simulink library "myLibrary"  (R2023a)
settings: Solver=VariableStepAuto  StartTime=0.0  StopTime=10.0  RelTol=1e-3
undefined symbols (not defined in the file): Cac_n1, ctrl1, Da, Discrete, dtha, ee_sli_rtmsupport, FA, gcbh, Ha, Ini, init_line, init_load, init_SG, init_TH, init_trafo, init_VSC, initMachineBlocks, Ka, Lf, Llkd_pu, Llkq1_pu, NET, P, plots_step, q0, Rac_n1, Radd, Rkd_pu, Rkq1_pu, Rload_add, sim_config, spsSteamTurbineModel, T_global, T_load, T_NET, T_SG, T_TH, T_trafo, T_VSC, Ts, tstep, V1
libraries: spsSeriesRLCBranchLib x57, spsParallelRLCBranchLib x39, eeGeneralControl x38, spsCurrentMeasurementLib x20, spsFirstOrderFilterLib x16, spsVoltageMeasurementLib x14, spsControlledVoltageSourceLib x12, $bdroot x9, dspsigops x6, spsThreePhaseVIMeasurementLib x5, spsPLL3phLib x4, spsThreePhaseBreakerLib x3
(part 5 of 7)

== system myLibrary/GFOL/Control/Is3/Matriu T ==
  u : Inport
  Constant : Constant  Value=(2/3)*[1/2 1/2 1/2]
  Fcn : Fcn  Expr=(2/3)*cos(u)
  Fcn1 : Fcn  Expr=(2/3)*cos(u-(2*pi)/3)
  Fcn2 : Fcn  Expr=(2/3)*cos(u+(2*pi)/3)
  Fcn3 : Fcn  Expr=(2/3)*sin(u)
  Fcn4 : Fcn  Expr=(2/3)*sin(u-(2*pi)/3)
  Fcn5 : Fcn  Expr=(2/3)*sin(u+(2*pi)/3)
  Math Function : Math  Operator=transpose  SignedPower=on
  Matrix Concatenate : Concatenate  NumInputs=3  Mode=Multidimensional array  ConcatenateDimension=2
  Mux : Mux  Inputs=3
  Mux1 : Mux  Inputs=3
  Out1 : Outport  VectorParamsAs1DForOutWhenUnconnected=off
  wires:
  u/1 -> Fcn/1, Fcn1/1, Fcn2/1, Fcn3/1, Fcn4/1, Fcn5/1
  Fcn3/1 -> Mux1/1
  Fcn4/1 -> Mux1/2
  Fcn5/1 -> Mux1/3
  Mux/1 -> Matrix Concatenate/1
  Constant/1 -> Matrix Concatenate/3
  Fcn/1 -> Mux/1
  Fcn1/1 -> Mux/2
  Fcn2/1 -> Mux/3
  Mux1/1 -> Matrix Concatenate/2
  Matrix Concatenate/1 -> Math Function/1
  Math Function/1 -> Out1/1

== system myLibrary/GFOL/Control/Is4/Matriu T ==
  u : Inport
  Constant : Constant  Value=(2/3)*[1/2 1/2 1/2]
  Fcn : Fcn  Expr=(2/3)*cos(u)
  Fcn1 : Fcn  Expr=(2/3)*cos(u-(2*pi)/3)
  Fcn2 : Fcn  Expr=(2/3)*cos(u+(2*pi)/3)
  Fcn3 : Fcn  Expr=(2/3)*sin(u)
  Fcn4 : Fcn  Expr=(2/3)*sin(u-(2*pi)/3)
  Fcn5 : Fcn  Expr=(2/3)*sin(u+(2*pi)/3)
  Math Function : Math  Operator=transpose  SignedPower=on
  Matrix Concatenate : Concatenate  NumInputs=3  Mode=Multidimensional array  ConcatenateDimension=2
  Mux : Mux  Inputs=3
  Mux1 : Mux  Inputs=3
  Out1 : Outport  VectorParamsAs1DForOutWhenUnconnected=off
  wires:
  Math Function/1 -> Out1/1
  Matrix Concatenate/1 -> Math Function/1
  Mux1/1 -> Matrix Concatenate/2
  Fcn2/1 -> Mux/3
  Fcn1/1 -> Mux/2
  Fcn/1 -> Mux/1
  Constant/1 -> Matrix Concatenate/3
  Mux/1 -> Matrix Concatenate/1
  Fcn5/1 -> Mux1/3
  Fcn4/1 -> Mux1/2
  Fcn3/1 -> Mux1/1
  u/1 -> Fcn5/1, Fcn4/1, Fcn3/1, Fcn2/1, Fcn1/1, Fcn/1

== system myLibrary/GFOL/Control/Is5/Matriu T ==
  u : Inport
  Constant : Constant  Value=(2/3)*[1/2 1/2 1/2]
  Fcn : Fcn  Expr=(2/3)*cos(u)
  Fcn1 : Fcn  Expr=(2/3)*cos(u-(2*pi)/3)
  Fcn2 : Fcn  Expr=(2/3)*cos(u+(2*pi)/3)
  Fcn3 : Fcn  Expr=(2/3)*sin(u)
  Fcn4 : Fcn  Expr=(2/3)*sin(u-(2*pi)/3)
  Fcn5 : Fcn  Expr=(2/3)*sin(u+(2*pi)/3)
  Math Function : Math  Operator=transpose  SignedPower=on
  Matrix Concatenate : Concatenate  NumInputs=3  Mode=Multidimensional array  ConcatenateDimension=2
  Mux : Mux  Inputs=3
  Mux1 : Mux  Inputs=3
  Out1 : Outport  VectorParamsAs1DForOutWhenUnconnected=off
  wires:
  u/1 -> Fcn/1, Fcn1/1, Fcn2/1, Fcn3/1, Fcn4/1, Fcn5/1
  Fcn3/1 -> Mux1/1
  Fcn4/1 -> Mux1/2
  Fcn5/1 -> Mux1/3
  Mux/1 -> Matrix Concatenate/1
  Constant/1 -> Matrix Concatenate/3
  Fcn/1 -> Mux/1
  Fcn1/1 -> Mux/2
  Fcn2/1 -> Mux/3
  Mux1/1 -> Matrix Concatenate/2
  Matrix Concatenate/1 -> Math Function/1
  Math Function/1 -> Out1/1

== system myLibrary/GFOL/Control/Is7/Matriu T ==
  u : Inport
  Constant : Constant  Value=(2/3)*[1/2 1/2 1/2]
  Fcn : Fcn  Expr=(2/3)*cos(u)
  Fcn1 : Fcn  Expr=(2/3)*cos(u-(2*pi)/3)
  Fcn2 : Fcn  Expr=(2/3)*cos(u+(2*pi)/3)
  Fcn3 : Fcn  Expr=(2/3)*sin(u)
  Fcn4 : Fcn  Expr=(2/3)*sin(u-(2*pi)/3)
  Fcn5 : Fcn  Expr=(2/3)*sin(u+(2*pi)/3)
  Math Function : Math  Operator=transpose  SignedPower=on
  Matrix Concatenate : Concatenate  NumInputs=3  Mode=Multidimensional array  ConcatenateDimension=2
  Mux : Mux  Inputs=3
  Mux1 : Mux  Inputs=3
  Out1 : Outport  VectorParamsAs1DForOutWhenUnconnected=off
  wires:
  Math Function/1 -> Out1/1
  Matrix Concatenate/1 -> Math Function/1
  Mux1/1 -> Matrix Concatenate/2
  Fcn2/1 -> Mux/3
  Fcn1/1 -> Mux/2
  Fcn/1 -> Mux/1
  Constant/1 -> Matrix Concatenate/3
  Mux/1 -> Matrix Concatenate/1
  Fcn5/1 -> Mux1/3
  Fcn4/1 -> Mux1/2
  Fcn3/1 -> Mux1/1
  u/1 -> Fcn5/1, Fcn4/1, Fcn3/1, Fcn2/1, Fcn1/1, Fcn/1

== system myLibrary/GFOL/Control/PLL/Tpark ==
  Va : Inport
  Vb : Inport  Port=2
  Vc : Inport  Port=3
  u : Inport  Port=4
  Demux : Demux  Outputs=3
  Matriu T : Subsystem
  Mux : Mux  Inputs=3
      settings: DisplayOption=signals
  Product : Product  Multiplication=Matrix(*)
  Vq : Outport  VectorParamsAs1DForOutWhenUnconnected=off
  Vd : Outport  Port=2  VectorParamsAs1DForOutWhenUnconnected=off
  0 : Outport  Port=3  VectorParamsAs1DForOutWhenUnconnected=off
  wires:
  Matriu T/1(Out1) -> Product/1
  Mux/1 -> Product/2
  u/1 -> Matriu T/1(u)
  Demux/3 -> 0/1
  Demux/2 -> Vd/1
  Demux/1 -> Vq/1
  Product/1 -> Demux/1
  Vc/1 -> Mux/3
  Vb/1 -> Mux/2
  Va/1 -> Mux/1

== system myLibrary/GFOL_RL/Control/Is/Matriu T ==
  u : Inport
  Constant : Constant  Value=(2/3)*[1/2 1/2 1/2]
  Fcn : Fcn  Expr=(2/3)*cos(u)
  Fcn1 : Fcn  Expr=(2/3)*cos(u-(2*pi)/3)
  Fcn2 : Fcn  Expr=(2/3)*cos(u+(2*pi)/3)
  Fcn3 : Fcn  Expr=(2/3)*sin(u)
  Fcn4 : Fcn  Expr=(2/3)*sin(u-(2*pi)/3)
  Fcn5 : Fcn  Expr=(2/3)*sin(u+(2*pi)/3)
  Math Function : Math  Operator=transpose  SignedPower=on
  Matrix Concatenate : Concatenate  NumInputs=3  Mode=Multidimensional array  ConcatenateDimension=2
  Mux : Mux  Inputs=3
  Mux1 : Mux  Inputs=3
  Out1 : Outport  VectorParamsAs1DForOutWhenUnconnected=off
  wires:
  u/1 -> Fcn/1, Fcn1/1, Fcn2/1, Fcn3/1, Fcn4/1, Fcn5/1
  Fcn3/1 -> Mux1/1
  Fcn4/1 -> Mux1/2
  Fcn5/1 -> Mux1/3
  Mux/1 -> Matrix Concatenate/1
  Constant/1 -> Matrix Concatenate/3
  Fcn/1 -> Mux/1
  Fcn1/1 -> Mux/2
  Fcn2/1 -> Mux/3
  Mux1/1 -> Matrix Concatenate/2
  Matrix Concatenate/1 -> Math Function/1
  Math Function/1 -> Out1/1

== system myLibrary/GFOL_RL/Control/Is1/Matriu T ==
  u : Inport
  Constant : Constant  Value=(2/3)*[1/2 1/2 1/2]
  Fcn : Fcn  Expr=(2/3)*cos(u)
  Fcn1 : Fcn  Expr=(2/3)*cos(u-(2*pi)/3)
  Fcn2 : Fcn  Expr=(2/3)*cos(u+(2*pi)/3)
  Fcn3 : Fcn  Expr=(2/3)*sin(u)
  Fcn4 : Fcn  Expr=(2/3)*sin(u-(2*pi)/3)
  Fcn5 : Fcn  Expr=(2/3)*sin(u+(2*pi)/3)
  Math Function : Math  Operator=transpose  SignedPower=on
  Matrix Concatenate : Concatenate  NumInputs=3  Mode=Multidimensional array  ConcatenateDimension=2
  Mux : Mux  Inputs=3
  Mux1 : Mux  Inputs=3
  Out1 : Outport  VectorParamsAs1DForOutWhenUnconnected=off
  wires:
  Math Function/1 -> Out1/1
  Matrix Concatenate/1 -> Math Function/1
  Mux1/1 -> Matrix Concatenate/2
  Fcn2/1 -> Mux/3
  Fcn1/1 -> Mux/2
  Fcn/1 -> Mux/1
  Constant/1 -> Matrix Concatenate/3
  Mux/1 -> Matrix Concatenate/1
  Fcn5/1 -> Mux1/3
  Fcn4/1 -> Mux1/2
  Fcn3/1 -> Mux1/1
  u/1 -> Fcn5/1, Fcn4/1, Fcn3/1, Fcn2/1, Fcn1/1, Fcn/1

== system myLibrary/GFOL_RL/Control/Is3/Matriu T ==
  u : Inport
  Constant : Constant  Value=(2/3)*[1/2 1/2 1/2]
  Fcn : Fcn  Expr=(2/3)*cos(u)
  Fcn1 : Fcn  Expr=(2/3)*cos(u-(2*pi)/3)
  Fcn2 : Fcn  Expr=(2/3)*cos(u+(2*pi)/3)
  Fcn3 : Fcn  Expr=(2/3)*sin(u)
  Fcn4 : Fcn  Expr=(2/3)*sin(u-(2*pi)/3)
  Fcn5 : Fcn  Expr=(2/3)*sin(u+(2*pi)/3)
  Math Function : Math  Operator=transpose  SignedPower=on
  Matrix Concatenate : Concatenate  NumInputs=3  Mode=Multidimensional array  ConcatenateDimension=2
  Mux : Mux  Inputs=3
  Mux1 : Mux  Inputs=3
  Out1 : Outport  VectorParamsAs1DForOutWhenUnconnected=off
  wires:
  u/1 -> Fcn/1, Fcn1/1, Fcn2/1, Fcn3/1, Fcn4/1, Fcn5/1
  Fcn3/1 -> Mux1/1
  Fcn4/1 -> Mux1/2
  Fcn5/1 -> Mux1/3
  Mux/1 -> Matrix Concatenate/1
  Constant/1 -> Matrix Concatenate/3
  Fcn/1 -> Mux/1
  Fcn1/1 -> Mux/2
  Fcn2/1 -> Mux/3
  Mux1/1 -> Matrix Concatenate/2
  Matrix Concatenate/1 -> Math Function/1
  Math Function/1 -> Out1/1

== system myLibrary/GFOL_RL/Control/Is4/Matriu T ==
  u : Inport
  Constant : Constant  Value=(2/3)*[1/2 1/2 1/2]
  Fcn : Fcn  Expr=(2/3)*cos(u)
  Fcn1 : Fcn  Expr=(2/3)*cos(u-(2*pi)/3)
  Fcn2 : Fcn  Expr=(2/3)*cos(u+(2*pi)/3)
  Fcn3 : Fcn  Expr=(2/3)*sin(u)
  Fcn4 : Fcn  Expr=(2/3)*sin(u-(2*pi)/3)
  Fcn5 : Fcn  Expr=(2/3)*sin(u+(2*pi)/3)
  Math Function : Math  Operator=transpose  SignedPower=on
  Matrix Concatenate : Concatenate  NumInputs=3  Mode=Multidimensional array  ConcatenateDimension=2
  Mux : Mux  Inputs=3
  Mux1 : Mux  Inputs=3
  Out1 : Outport  VectorParamsAs1DForOutWhenUnconnected=off
  wires:
  Math Function/1 -> Out1/1
  Matrix Concatenate/1 -> Math Function/1
  Mux1/1 -> Matrix Concatenate/2
  Fcn2/1 -> Mux/3
  Fcn1/1 -> Mux/2
  Fcn/1 -> Mux/1
  Constant/1 -> Matrix Concatenate/3
  Mux/1 -> Matrix Concatenate/1
  Fcn5/1 -> Mux1/3
  Fcn4/1 -> Mux1/2
  Fcn3/1 -> Mux1/1
  u/1 -> Fcn5/1, Fcn4/1, Fcn3/1, Fcn2/1, Fcn1/1, Fcn/1

== system myLibrary/GFOL_RL/Control/Is5/Matriu T ==
  u : Inport
  Constant : Constant  Value=(2/3)*[1/2 1/2 1/2]
  Fcn : Fcn  Expr=(2/3)*cos(u)
  Fcn1 : Fcn  Expr=(2/3)*cos(u-(2*pi)/3)
  Fcn2 : Fcn  Expr=(2/3)*cos(u+(2*pi)/3)
  Fcn3 : Fcn  Expr=(2/3)*sin(u)
  Fcn4 : Fcn  Expr=(2/3)*sin(u-(2*pi)/3)
  Fcn5 : Fcn  Expr=(2/3)*sin(u+(2*pi)/3)
  Math Function : Math  Operator=transpose  SignedPower=on
  Matrix Concatenate : Concatenate  NumInputs=3  Mode=Multidimensional array  ConcatenateDimension=2
  Mux : Mux  Inputs=3
  Mux1 : Mux  Inputs=3
  Out1 : Outport  VectorParamsAs1DForOutWhenUnconnected=off
  wires:
  u/1 -> Fcn/1, Fcn1/1, Fcn2/1, Fcn3/1, Fcn4/1, Fcn5/1
  Fcn3/1 -> Mux1/1
  Fcn4/1 -> Mux1/2
  Fcn5/1 -> Mux1/3
  Mux/1 -> Matrix Concatenate/1
  Constant/1 -> Matrix Concatenate/3
  Fcn/1 -> Mux/1
  Fcn1/1 -> Mux/2
  Fcn2/1 -> Mux/3
  Mux1/1 -> Matrix Concatenate/2
  Matrix Concatenate/1 -> Math Function/1
  Math Function/1 -> Out1/1

== system myLibrary/GFOL_RL/Control/PLL/Tpark ==
  Va : Inport
  Vb : Inport  Port=2
  Vc : Inport  Port=3
  u : Inport  Port=4
  Demux : Demux  Outputs=3
  Matriu T : Subsystem
  Mux : Mux  Inputs=3
      settings: DisplayOption=signals
  Product : Product  Multiplication=Matrix(*)
  Vq : Outport  VectorParamsAs1DForOutWhenUnconnected=off
  Vd : Outport  Port=2  VectorParamsAs1DForOutWhenUnconnected=off
  0 : Outport  Port=3  VectorParamsAs1DForOutWhenUnconnected=off
  wires:
  Matriu T/1(Out1) -> Product/1
  Mux/1 -> Product/2
  u/1 -> Matriu T/1(u)
  Demux/3 -> 0/1
  Demux/2 -> Vd/1
  Demux/1 -> Vq/1
  Product/1 -> Demux/1
  Vc/1 -> Mux/3
  Vb/1 -> Mux/2
  Va/1 -> Mux/1

== system myLibrary/GFOR/Control/Is/Matriu T ==
  u : Inport
  Constant : Constant  Value=(2/3)*[1/2 1/2 1/2]
  Fcn : Fcn  Expr=(2/3)*cos(u)
  Fcn1 : Fcn  Expr=(2/3)*cos(u-(2*pi)/3)
  Fcn2 : Fcn  Expr=(2/3)*cos(u+(2*pi)/3)
  Fcn3 : Fcn  Expr=(2/3)*sin(u)
  Fcn4 : Fcn  Expr=(2/3)*sin(u-(2*pi)/3)
  Fcn5 : Fcn  Expr=(2/3)*sin(u+(2*pi)/3)
  Math Function : Math  Operator=transpose  SignedPower=on
  Matrix Concatenate : Concatenate  NumInputs=3  Mode=Multidimensional array  ConcatenateDimension=2
  Mux : Mux  Inputs=3
  Mux1 : Mux  Inputs=3
  Out1 : Outport  VectorParamsAs1DForOutWhenUnconnected=off
  wires:
  Math Function/1 -> Out1/1
  Matrix Concatenate/1 -> Math Function/1
  Mux1/1 -> Matrix Concatenate/2
  Fcn2/1 -> Mux/3
  Fcn1/1 -> Mux/2
  Fcn/1 -> Mux/1
  Constant/1 -> Matrix Concatenate/3
  Mux/1 -> Matrix Concatenate/1
  Fcn5/1 -> Mux1/3
  Fcn4/1 -> Mux1/2
  Fcn3/1 -> Mux1/1
  u/1 -> Fcn5/1, Fcn4/1, Fcn3/1, Fcn2/1, Fcn1/1, Fcn/1

== system myLibrary/GFOR/Control/Is2/Matriu T ==
  u : Inport
  Constant : Constant  Value=(2/3)*[1/2 1/2 1/2]
  Fcn : Fcn  Expr=(2/3)*cos(u)
  Fcn1 : Fcn  Expr=(2/3)*cos(u-(2*pi)/3)
  Fcn2 : Fcn  Expr=(2/3)*cos(u+(2*pi)/3)
  Fcn3 : Fcn  Expr=(2/3)*sin(u)
  Fcn4 : Fcn  Expr=(2/3)*sin(u-(2*pi)/3)
  Fcn5 : Fcn  Expr=(2/3)*sin(u+(2*pi)/3)
  Math Function : Math  Operator=transpose  SignedPower=on
  Matrix Concatenate : Concatenate  NumInputs=3  Mode=Multidimensional array  ConcatenateDimension=2
  Mux : Mux  Inputs=3
  Mux1 : Mux  Inputs=3
  Out1 : Outport  VectorParamsAs1DForOutWhenUnconnected=off
  wires:
  Math Function/1 -> Out1/1
  Matrix Concatenate/1 -> Math Function/1
  Mux1/1 -> Matrix Concatenate/2
  Fcn2/1 -> Mux/3
  Fcn1/1 -> Mux/2
  Fcn/1 -> Mux/1
  Constant/1 -> Matrix Concatenate/3
  Mux/1 -> Matrix Concatenate/1
  Fcn5/1 -> Mux1/3
  Fcn4/1 -> Mux1/2
  Fcn3/1 -> Mux1/1
  u/1 -> Fcn5/1, Fcn4/1, Fcn3/1, Fcn2/1, Fcn1/1, Fcn/1

== system myLibrary/SG/Exciter/Exciter ST4B/Fex ==
  V_E : Inport
  Ifd : Inport  Port=2
  Data Type Conversion Inherited : simulink/Signal Attributes/Data Type Conversion Inherited  ConvertRealWorld=Real World Value  DoSatur=off
  Divide : Product  Inputs=*/
  Gain : Gain  Gain=K_C  OutDataTypeStr=double
  Prevent divide by zero : Fcn  Expr=u+(u==0)*eps
  fex : MATLAB Function  TreatAsAtomicUnit=on
  F_EX : Outport  VectorParamsAs1DForOutWhenUnconnected=off
  wires:
  Data Type Conversion Inherited/1 -> F_EX/1
  fex/1(F_EX) -> Data Type Conversion Inherited/2  "F_EX"
  Gain/1 -> fex/1(I_N)  "I_N"
  Divide/1 -> Gain/1
  V_E/1 -> Prevent divide by zero/1
  Ifd/1 -> Divide/1, Data Type Conversion Inherited/1
  Prevent divide by zero/1 -> Divide/2

== system myLibrary/SG/Exciter/Exciter ST4B/PI_M ==
  u : Inport
  Constant2 : Constant  Value=0
  Gain2 : Gain  Gain=K_PM
  Gain3 : Gain  Gain=K_IM
  Integrator (Discrete or Continuous) : eeGeneralControl/Integrator (Discrete or Continuous)  LabelModeActiveChoice=Discrete  ExternalReset=level  LimitType=Anti-windup  B=inf  A=-inf  Ts=Ts
  Sum6 : Sum
  y : Outport
  wires:
  Gain3/1 -> Integrator (Discrete or Continuous)/1, Integrator (Discrete or Continuous)/3
  u/1 -> Gain2/1, Gain3/1
  Constant2/1 -> Integrator (Discrete or Continuous)/2
  Integrator (Discrete or Continuous)/1 -> Sum6/2
  Gain2/1 -> Sum6/1
  Sum6/1 -> y/1

== system myLibrary/SG/Exciter/Exciter ST4B/PI_R ==
  u : Inport
  Constant2 : Constant  Value=0
  Gain2 : Gain  Gain=K_PR
  Gain3 : Gain  Gain=K_IR
  Integrator (Discrete or Continuous) : eeGeneralControl/Integrator (Discrete or Continuous)  LabelModeActiveChoice=Discrete  ExternalReset=level  LimitType=Anti-windup  B=inf  A=-inf  Ts=Ts
  Sum6 : Sum
  y : Outport
  wires:
  Gain3/1 -> Integrator (Discrete or Continuous)/1, Integrator (Discrete or Continuous)/3
  u/1 -> Gain2/1, Gain3/1
  Constant2/1 -> Integrator (Discrete or Continuous)/2
  Integrator (Discrete or Continuous)/1 -> Sum6/2
  Gain2/1 -> Sum6/1
  Sum6/1 -> y/1

== system myLibrary/SG/Exciter/Exciter ST4B/Subsystem1 ==
  V_T : Inport
  Gain1 : Gain  Gain=K_P
  Sqrt : Sqrt
  y : Outport
  wires:
  Gain1/1 -> Sqrt/1
  Sqrt/1 -> y/1
  V_T/1 -> Gain1/1

== system myLibrary/SG/Governor-Turbine/Steam Turbine and Governor/Model ==
  Pref : Inport
  wref : Inport  Port=2
  d_theta : Inport  Port=3
  wm : Inport  Port=4
  4 mass shaft : Subsystem  TreatAsAtomicUnit=on
  Constant3 : Constant  Value=T_SG.genType ~= 1
  Product : Product  InputSameDT=on  SaturateOnIntegerOverflow=on  OutDataTypeStr=Inherit: Same as first input
  Sum : Sum  Inputs=+  InputSameDT=on  SaturateOnIntegerOverflow=on  OutDataTypeStr=Inherit: Same as first input
  Switch1 : Switch  Threshold=0.5  SaturateOnIntegerOverflow=off
  Terminator1 : Terminator
  governor : Subsystem  mask(Speed regulator for thermal turbine){Rp=reg1(2)}
      mask prompts: Rp "Permanent droop Rp:"
  multi-mass : Constant  Value=T_SG.genType == 1
  steam turbine MM : Subsystem  mask(Thermal turbine){Fa=FA, Ta=turb1, f0=q0}
      mask prompts: Fa "Generator 1 torque fractions [ F1  F2  F3  F4 ]:"; Ta "Time constants [ T1  T2  T3  T4 ] (s):"; f0 "Initial flows f0:"
      mask init:
      | F2=Fa(1); F3=Fa(2); F4=Fa(3); F5=Fa(4);
      | if Ta(1)==0, T1=1; else T1=Ta(1); end; if Ta(2)==0, T2=1; else T2=Ta(2); end
      | if Ta(3)==0, T3=1; else T3=Ta(3); end; if Ta(4)==0, T4=1; else T4=Ta(4); end
  steam turbine SM : Subsystem  mask(Thermal turbine){Fa=FA, Ta=turb1, f0=q0}
      mask prompts: Fa "Generator 1 torque fractions [ F1  F2  F3  F4 ]:"; Ta "Time constants [ T1  T2  T3  T4 ] (s):"; f0 "Initial flows f0:"
      mask init:
      | F2=Fa(1); F3=Fa(2); F4=Fa(3); F5=Fa(4);
      | if Ta(1)==0, T1=1; else T1=Ta(1); end; if Ta(2)==0, T2=1; else T2=Ta(2); end
      | if Ta(3)==0, T3=1; else T3=Ta(3); end; if Ta(4)==0, T4=1; else T4=Ta(4); end
  Pm : Outport
  Tr5-2 : Outport  Port=2
  dw_5-2 : Outport  Port=3
  gate : Outport  Port=4
  wires:
  steam turbine SM/1(Tturb) -> Sum/1
  steam turbine MM/2(T5-2) -> 4 mass shaft/1(T5-2)
  governor/1(gate opening) -> gate/1, steam turbine MM/1(gate), steam turbine SM/1(gate)
  steam turbine MM/1(flowHp) -> Terminator1/1
  4 mass shaft/3(dw_5-2) -> dw_5-2/1
  d_theta/1 -> 4 mass shaft/2(d_theta)
  Constant3/1 -> Switch1/2
  Sum/1 -> Switch1/1
  4 mass shaft/1(Tm_g) -> Switch1/3
  Switch1/1 -> Product/1
  4 mass shaft/2(Tr2-5) -> Tr5-2/1
  Product/1 -> Pm/1
  wref/1 -> governor/2(wref)
  Pref/1 -> governor/1(Pref)
  wm/1 -> Product/2, governor/3(w)
  multi-mass/1 -> 4 mass shaft/Enable

== system myLibrary/SG_step/Exciter/Exciter ST4B/Fex ==
  V_E : Inport
  Ifd : Inport  Port=2
  Data Type Conversion Inherited : simulink/Signal Attributes/Data Type Conversion Inherited  ConvertRealWorld=Real World Value  DoSatur=off
  Divide : Product  Inputs=*/
  Gain : Gain  Gain=K_C  OutDataTypeStr=double
  Prevent divide by zero : Fcn  Expr=u+(u==0)*eps
  fex : MATLAB Function  TreatAsAtomicUnit=on
  F_EX : Outport  VectorParamsAs1DForOutWhenUnconnected=off
  wires:
  Data Type Conversion Inherited/1 -> F_EX/1
  fex/1(F_EX) -> Data Type Conversion Inherited/2  "F_EX"
  Gain/1 -> fex/1(I_N)  "I_N"
  Divide/1 -> Gain/1
  V_E/1 -> Prevent divide by zero/1
  Ifd/1 -> Divide/1, Data Type Conversion Inherited/1
  Prevent divide by zero/1 -> Divide/2

== system myLibrary/SG_step/Exciter/Exciter ST4B/PI_M ==
  u : Inport
  Constant2 : Constant  Value=0
  Gain2 : Gain  Gain=K_PM
  Gain3 : Gain  Gain=K_IM
  Integrator (Discrete or Continuous) : eeGeneralControl/Integrator (Discrete or Continuous)  LabelModeActiveChoice=Discrete  ExternalReset=level  LimitType=Anti-windup  B=inf  A=-inf  Ts=Ts
  Sum6 : Sum
  y : Outport
  wires:
  Gain3/1 -> Integrator (Discrete or Continuous)/1, Integrator (Discrete or Continuous)/3
  u/1 -> Gain2/1, Gain3/1
  Constant2/1 -> Integrator (Discrete or Continuous)/2
  Integrator (Discrete or Continuous)/1 -> Sum6/2
  Gain2/1 -> Sum6/1
  Sum6/1 -> y/1

== system myLibrary/SG_step/Exciter/Exciter ST4B/PI_R ==
  u : Inport
  Constant2 : Constant  Value=0
  Gain2 : Gain  Gain=K_PR
  Gain3 : Gain  Gain=K_IR
  Integrator (Discrete or Continuous) : eeGeneralControl/Integrator (Discrete or Continuous)  LabelModeActiveChoice=Discrete  ExternalReset=level  LimitType=Anti-windup  B=inf  A=-inf  Ts=Ts
  Sum6 : Sum
  y : Outport
  wires:
  Gain3/1 -> Integrator (Discrete or Continuous)/1, Integrator (Discrete or Continuous)/3
  u/1 -> Gain2/1, Gain3/1
  Constant2/1 -> Integrator (Discrete or Continuous)/2
  Integrator (Discrete or Continuous)/1 -> Sum6/2
  Gain2/1 -> Sum6/1
  Sum6/1 -> y/1

== system myLibrary/SG_step/Exciter/Exciter ST4B/Subsystem1 ==
  V_T : Inport
  Gain1 : Gain  Gain=K_P
  Sqrt : Sqrt
  y : Outport
  wires:
  Gain1/1 -> Sqrt/1
  Sqrt/1 -> y/1
  V_T/1 -> Gain1/1

== system myLibrary/SG_step/Governor-Turbine/Steam Turbine and Governor/Model ==
  Pref : Inport
  wref : Inport  Port=2
  d_theta : Inport  Port=3
  wm : Inport  Port=4
  4 mass shaft : Subsystem  TreatAsAtomicUnit=on
  Constant3 : Constant  Value=T_SG.genType ~= 1
  Product : Product  InputSameDT=on  SaturateOnIntegerOverflow=on  OutDataTypeStr=Inherit: Same as first input
  Sum : Sum  Inputs=+  InputSameDT=on  SaturateOnIntegerOverflow=on  OutDataTypeStr=Inherit: Same as first input
  Switch1 : Switch  Threshold=0.5  SaturateOnIntegerOverflow=off
  Terminator1 : Terminator
  governor : Subsystem  mask(Speed regulator for thermal turbine){Rp=reg1(2)}
      mask prompts: Rp "Permanent droop Rp:"
  multi-mass : Constant  Value=T_SG.genType == 1
  steam turbine MM : Subsystem  mask(Thermal turbine){Fa=FA, Ta=turb1, f0=q0}
      mask prompts: Fa "Generator 1 torque fractions [ F1  F2  F3  F4 ]:"; Ta "Time constants [ T1  T2  T3  T4 ] (s):"; f0 "Initial flows f0:"
      mask init:
      | F2=Fa(1); F3=Fa(2); F4=Fa(3); F5=Fa(4);
      | if Ta(1)==0, T1=1; else T1=Ta(1); end; if Ta(2)==0, T2=1; else T2=Ta(2); end
      | if Ta(3)==0, T3=1; else T3=Ta(3); end; if Ta(4)==0, T4=1; else T4=Ta(4); end
  steam turbine SM : Subsystem  mask(Thermal turbine){Fa=FA, Ta=turb1, f0=q0}
      mask prompts: Fa "Generator 1 torque fractions [ F1  F2  F3  F4 ]:"; Ta "Time constants [ T1  T2  T3  T4 ] (s):"; f0 "Initial flows f0:"
      mask init:
      | F2=Fa(1); F3=Fa(2); F4=Fa(3); F5=Fa(4);
      | if Ta(1)==0, T1=1; else T1=Ta(1); end; if Ta(2)==0, T2=1; else T2=Ta(2); end
      | if Ta(3)==0, T3=1; else T3=Ta(3); end; if Ta(4)==0, T4=1; else T4=Ta(4); end
  Pm : Outport
  Tr5-2 : Outport  Port=2
  dw_5-2 : Outport  Port=3
  gate : Outport  Port=4
  wires:
  steam turbine SM/1(Tturb) -> Sum/1
  steam turbine MM/2(T5-2) -> 4 mass shaft/1(T5-2)
  governor/1(gate opening) -> gate/1, steam turbine MM/1(gate), steam turbine SM/1(gate)
  steam turbine MM/1(flowHp) -> Terminator1/1
  4 mass shaft/3(dw_5-2) -> dw_5-2/1
  d_theta/1 -> 4 mass shaft/2(d_theta)
  Constant3/1 -> Switch1/2
  Sum/1 -> Switch1/1
  4 mass shaft/1(Tm_g) -> Switch1/3
  Switch1/1 -> Product/1
  4 mass shaft/2(Tr2-5) -> Tr5-2/1
  Product/1 -> Pm/1
  wref/1 -> governor/2(wref)
  Pref/1 -> governor/1(Pref)
  wm/1 -> Product/2, governor/3(w)
  multi-mass/1 -> 4 mass shaft/Enable

== system myLibrary/GFOL/Control/PLL/Tpark/Matriu T ==
  u : Inport
  Constant : Constant  Value=(2/3)*[1/2 1/2 1/2]
  Fcn : Fcn  Expr=(2/3)*cos(u)
  Fcn1 : Fcn  Expr=(2/3)*cos(u-(2*pi)/3)
  Fcn2 : Fcn  Expr=(2/3)*cos(u+(2*pi)/3)
  Fcn3 : Fcn  Expr=(2/3)*sin(u)
  Fcn4 : Fcn  Expr=(2/3)*sin(u-(2*pi)/3)
  Fcn5 : Fcn  Expr=(2/3)*sin(u+(2*pi)/3)
  Math Function : Math  Operator=transpose  SignedPower=on
  Matrix Concatenate : Concatenate  NumInputs=3  Mode=Multidimensional array  ConcatenateDimension=2
  Mux : Mux  Inputs=3
  Mux1 : Mux  Inputs=3
  Out1 : Outport  VectorParamsAs1DForOutWhenUnconnected=off
  wires:
  Math Function/1 -> Out1/1
  Matrix Concatenate/1 -> Math Function/1
  Mux1/1 -> Matrix Concatenate/2
  Fcn2/1 -> Mux/3
  Fcn1/1 -> Mux/2
  Fcn/1 -> Mux/1
  Constant/1 -> Matrix Concatenate/3
  Mux/1 -> Matrix Concatenate/1
  Fcn5/1 -> Mux1/3
  Fcn4/1 -> Mux1/2
  Fcn3/1 -> Mux1/1
  u/1 -> Fcn/1, Fcn1/1, Fcn2/1, Fcn3/1, Fcn4/1, Fcn5/1

== system myLibrary/GFOL_RL/Control/PLL/Tpark/Matriu T ==
  u : Inport
  Constant : Constant  Value=(2/3)*[1/2 1/2 1/2]
  Fcn : Fcn  Expr=(2/3)*cos(u)
  Fcn1 : Fcn  Expr=(2/3)*cos(u-(2*pi)/3)
  Fcn2 : Fcn  Expr=(2/3)*cos(u+(2*pi)/3)
  Fcn3 : Fcn  Expr=(2/3)*sin(u)
  Fcn4 : Fcn  Expr=(2/3)*sin(u-(2*pi)/3)
  Fcn5 : Fcn  Expr=(2/3)*sin(u+(2*pi)/3)
  Math Function : Math  Operator=transpose  SignedPower=on
  Matrix Concatenate : Concatenate  NumInputs=3  Mode=Multidimensional array  ConcatenateDimension=2
  Mux : Mux  Inputs=3
  Mux1 : Mux  Inputs=3
  Out1 : Outport  VectorParamsAs1DForOutWhenUnconnected=off
  wires:
  Math Function/1 -> Out1/1
  Matrix Concatenate/1 -> Math Function/1
  Mux1/1 -> Matrix Concatenate/2
  Fcn2/1 -> Mux/3
  Fcn1/1 -> Mux/2
  Fcn/1 -> Mux/1
  Constant/1 -> Matrix Concatenate/3
  Mux/1 -> Matrix Concatenate/1
  Fcn5/1 -> Mux1/3
  Fcn4/1 -> Mux1/2
  Fcn3/1 -> Mux1/1
  u/1 -> Fcn/1, Fcn1/1, Fcn2/1, Fcn3/1, Fcn4/1, Fcn5/1

== system myLibrary/SG/Governor-Turbine/Steam Turbine and Governor/Model/4 mass shaft ==
  T5-2 : Inport
  d_theta : Inport  Port=2
  Enable : EnablePort  PropagateVarSize=During execution
  1 mass : Subsystem  TreatAsAtomicUnit=on
  2 masses : Subsystem  TreatAsAtomicUnit=on
  3 masses : Subsystem  TreatAsAtomicUnit=on
  4 masses : Subsystem  TreatAsAtomicUnit=on
  Multiport Switch1 : MultiPortSwitch  Inputs=4  SaturateOnIntegerOverflow=off
  Multiport Switch2 : MultiPortSwitch  Inputs=4  SaturateOnIntegerOverflow=off
  Multiport Switch3 : MultiPortSwitch  Inputs=4  SaturateOnIntegerOverflow=off
  ctrl2 : Constant  Value=ctrl1==4
  ctrl3 : Constant  Value=ctrl1==3
  ctrl4 : Constant  Value=ctrl1
  ctrl6 : Constant  Value=ctrl1==2
  ctrl7 : Constant  Value=ctrl1==1
  Tm_g : Outport  OutputWhenDisabled=reset  InitialOutput=0
  Tr2-5 : Outport  Port=2  OutputWhenDisabled=reset  InitialOutput=[0 0 0 0]
  dw_5-2 : Outport  Port=3  OutputWhenDisabled=reset  InitialOutput=[0 0 0 0]
  wires:
  4 masses/2(dw_5-2) -> Multiport Switch3/5
  Multiport Switch3/1 -> dw_5-2/1
  Multiport Switch2/1 -> Tm_g/1
  Multiport Switch1/1 -> Tr2-5/1
  3 masses/2(dw_5-2) -> Multiport Switch3/4
  ctrl6/1 -> 2 masses/Enable
  ctrl7/1 -> 1 mass/Enable
  2 masses/2(dw_5-2) -> Multiport Switch3/3
  1 mass/2(dw_5-2) -> Multiport Switch3/2
  ctrl3/1 -> 3 masses/Enable
  ctrl2/1 -> 4 masses/Enable
  4 masses/3(Tm_gen) -> Multiport Switch2/5
  3 masses/3(Tm_gen) -> Multiport Switch2/4
  2 masses/3(Tm_gen) -> Multiport Switch2/3
  ctrl4/1 -> Multiport Switch3/1, Multiport Switch2/1, Multiport Switch1/1
  1 mass/3(Tm_gen) -> Multiport Switch2/2
  d_theta/1 -> 4 masses/2(dth_gen), 3 masses/2(dth_gen), 2 masses/2(dth_gen), 1 mass/2(dth_gen)
  T5-2/1 -> 4 masses/1(Tt_5-2), 3 masses/1(Tt_5-2), 2 masses/1(Tt_5-2), 1 mass/1(Tt_5-2)
  4 masses/1(Ts_5-2) -> Multiport Switch1/5
  3 masses/1(Ts_5-2) -> Multiport Switch1/4
  2 masses/1(Ts_5-2) -> Multiport Switch1/3
  1 mass/1(Ts_5-2) -> Multiport Switch1/2

== system myLibrary/SG/Governor-Turbine/Steam Turbine and Governor/Model/governor ==
  Pref : Inport
  wref : Inport  Port=2
  w : Inport  Port=3
  Gain : Gain  Gain=1/Rp  SaturateOnIntegerOverflow=on  OutDataTypeStr=Inherit: Same as input  ParamDataTypeStr=Inherit: Same as input
  Gain4 : Gain  Gain=1/Rp  SaturateOnIntegerOverflow=on  OutDataTypeStr=Inherit: Same as input  ParamDataTypeStr=Inherit: Same as input
  Sum3 : Sum  Inputs=++-  InputSameDT=on  SaturateOnIntegerOverflow=on  OutDataTypeStr=Inherit: Same as first input
  gate opening : Outport
  wires:
  wref/1 -> Gain4/1
  Sum3/1 -> gate opening/1
  w/1 -> Gain/1
  Gain/1 -> Sum3/3
  Pref/1 -> Sum3/1
  Gain4/1 -> Sum3/2

== system myLibrary/SG/Governor-Turbine/Steam Turbine and Governor/Model/steam turbine MM ==
  gate : Inport
  Gain : Gain  Gain=F2  SaturateOnIntegerOverflow=on  OutDataTypeStr=Inherit: Same as input  ParamDataTypeStr=Inherit: Same as input
  Gain2 : Gain  Gain=F3  SaturateOnIntegerOverflow=on  OutDataTypeStr=Inherit: Same as input  ParamDataTypeStr=Inherit: Same as input
  Gain3 : Gain  Gain=F4  SaturateOnIntegerOverflow=on  OutDataTypeStr=Inherit: Same as input  ParamDataTypeStr=Inherit: Same as input
  Gain4 : Gain  Gain=F5  SaturateOnIntegerOverflow=on  OutDataTypeStr=Inherit: Same as input  ParamDataTypeStr=Inherit: Same as input
  Mux : Mux
  Scope : Scope  NumInputPorts=4
  Stage 1 : Subsystem
  "Stage 2 " : Subsystem
  Stage 3 : Subsystem
  Stage 4 : Subsystem
  flowHp : Outport
  T5-2 : Outport  Port=2
  wires:
  Stage 4/1(Out1) -> Gain4/1, Stage 3/1(In1), Scope/2, flowHp/1
  gate/1 -> Stage 4/1(In1), Scope/1
  Stage 3/1(Out1) -> Gain3/1, "Stage 2 "/1(In1), Scope/3
  Gain4/1 -> Mux/1
  Gain3/1 -> Mux/2
  Gain2/1 -> Mux/3
  Gain/1 -> Mux/4
  "Stage 2 "/1(Out1) -> Gain2/1, Stage 1/1(In1), Scope/4
  Stage 1/1(Out1) -> Gain/1
  Mux/1 -> T5-2/1

== system myLibrary/SG/Governor-Turbine/Steam Turbine and Governor/Model/steam turbine SM ==
  gate : Inport
  Gain : Gain  Gain=(1-initMachineBlocks{SGnum,13}(1))
  Gain1 : Gain  Gain=initMachineBlocks{SGnum,13}(1)
  Stage4 : spsFirstOrderFilterLib/First-Order Filter  FilterType=Lowpass  Tc=initMachineBlocks{SGnum,13}(2)  Ts=Ts  Initialize=on  Vac_Init=[0, 0, T_SG.fb]  Vdc_Init=(1-initMachineBlocks{SGnum,13}(1))*initSG.Pm  PlotResponse=off  FreqRange="[0,  200,  1]"
  Sum : Sum  Inputs=++|
  Tturb : Outport
  wires:
  Stage4/1 -> Sum/2
  Gain1/1 -> Sum/1
  Sum/1 -> Tturb/1
  Gain/1 -> Stage4/1
  gate/1 -> Gain/1, Gain1/1

== system myLibrary/SG_step/Governor-Turbine/Steam Turbine and Governor/Model/4 mass shaft ==
  T5-2 : Inport
  d_theta : Inport  Port=2
  Enable : EnablePort  PropagateVarSize=During execution
  1 mass : Subsystem  TreatAsAtomicUnit=on
  2 masses : Subsystem  TreatAsAtomicUnit=on
  3 masses : Subsystem  TreatAsAtomicUnit=on
  4 masses : Subsystem  TreatAsAtomicUnit=on
  Multiport Switch1 : MultiPortSwitch  Inputs=4  SaturateOnIntegerOverflow=off
  Multiport Switch2 : MultiPortSwitch  Inputs=4  SaturateOnIntegerOverflow=off
  Multiport Switch3 : MultiPortSwitch  Inputs=4  SaturateOnIntegerOverflow=off
  ctrl2 : Constant  Value=ctrl1==4
  ctrl3 : Constant  Value=ctrl1==3
  ctrl4 : Constant  Value=ctrl1
  ctrl6 : Constant  Value=ctrl1==2
  ctrl7 : Constant  Value=ctrl1==1
  Tm_g : Outport  OutputWhenDisabled=reset  InitialOutput=0
  Tr2-5 : Outport  Port=2  OutputWhenDisabled=reset  InitialOutput=[0 0 0 0]
  dw_5-2 : Outport  Port=3  OutputWhenDisabled=reset  InitialOutput=[0 0 0 0]
  wires:
  4 masses/2(dw_5-2) -> Multiport Switch3/5
  Multiport Switch3/1 -> dw_5-2/1
  Multiport Switch2/1 -> Tm_g/1
  Multiport Switch1/1 -> Tr2-5/1
  3 masses/2(dw_5-2) -> Multiport Switch3/4
  ctrl6/1 -> 2 masses/Enable
  ctrl7/1 -> 1 mass/Enable
  2 masses/2(dw_5-2) -> Multiport Switch3/3
  1 mass/2(dw_5-2) -> Multiport Switch3/2
  ctrl3/1 -> 3 masses/Enable
  ctrl2/1 -> 4 masses/Enable
  4 masses/3(Tm_gen) -> Multiport Switch2/5
  3 masses/3(Tm_gen) -> Multiport Switch2/4
  2 masses/3(Tm_gen) -> Multiport Switch2/3
  ctrl4/1 -> Multiport Switch3/1, Multiport Switch2/1, Multiport Switch1/1
  1 mass/3(Tm_gen) -> Multiport Switch2/2
  d_theta/1 -> 4 masses/2(dth_gen), 3 masses/2(dth_gen), 2 masses/2(dth_gen), 1 mass/2(dth_gen)
  T5-2/1 -> 4 masses/1(Tt_5-2), 3 masses/1(Tt_5-2), 2 masses/1(Tt_5-2), 1 mass/1(Tt_5-2)
  4 masses/1(Ts_5-2) -> Multiport Switch1/5
  3 masses/1(Ts_5-2) -> Multiport Switch1/4
  2 masses/1(Ts_5-2) -> Multiport Switch1/3
  1 mass/1(Ts_5-2) -> Multiport Switch1/2

== system myLibrary/SG_step/Governor-Turbine/Steam Turbine and Governor/Model/governor ==
  Pref : Inport
  wref : Inport  Port=2
  w : Inport  Port=3
  Gain : Gain  Gain=1/Rp  SaturateOnIntegerOverflow=on  OutDataTypeStr=Inherit: Same as input  ParamDataTypeStr=Inherit: Same as input
  Gain4 : Gain  Gain=1/Rp  SaturateOnIntegerOverflow=on  OutDataTypeStr=Inherit: Same as input  ParamDataTypeStr=Inherit: Same as input
  Sum3 : Sum  Inputs=++-  InputSameDT=on  SaturateOnIntegerOverflow=on  OutDataTypeStr=Inherit: Same as first input
  gate opening : Outport
  wires:
  wref/1 -> Gain4/1
  Sum3/1 -> gate opening/1
  w/1 -> Gain/1
  Gain/1 -> Sum3/3
  Pref/1 -> Sum3/1
  Gain4/1 -> Sum3/2

== system myLibrary/SG_step/Governor-Turbine/Steam Turbine and Governor/Model/steam turbine MM ==
  gate : Inport
  Gain : Gain  Gain=F2  SaturateOnIntegerOverflow=on  OutDataTypeStr=Inherit: Same as input  ParamDataTypeStr=Inherit: Same as input
  Gain2 : Gain  Gain=F3  SaturateOnIntegerOverflow=on  OutDataTypeStr=Inherit: Same as input  ParamDataTypeStr=Inherit: Same as input
  Gain3 : Gain  Gain=F4  SaturateOnIntegerOverflow=on  OutDataTypeStr=Inherit: Same as input  ParamDataTypeStr=Inherit: Same as input
  Gain4 : Gain  Gain=F5  SaturateOnIntegerOverflow=on  OutDataTypeStr=Inherit: Same as input  ParamDataTypeStr=Inherit: Same as input
  Mux : Mux
  Scope : Scope  NumInputPorts=4
  Stage 1 : Subsystem
  "Stage 2 " : Subsystem
  Stage 3 : Subsystem
  Stage 4 : Subsystem
  flowHp : Outport
  T5-2 : Outport  Port=2
  wires:
  Stage 4/1(Out1) -> Gain4/1, Stage 3/1(In1), Scope/2, flowHp/1
  gate/1 -> Stage 4/1(In1), Scope/1
  Stage 3/1(Out1) -> Gain3/1, "Stage 2 "/1(In1), Scope/3
  Gain4/1 -> Mux/1
  Gain3/1 -> Mux/2
  Gain2/1 -> Mux/3
  Gain/1 -> Mux/4
  "Stage 2 "/1(Out1) -> Gain2/1, Stage 1/1(In1), Scope/4
  Stage 1/1(Out1) -> Gain/1
  Mux/1 -> T5-2/1

== system myLibrary/SG_step/Governor-Turbine/Steam Turbine and Governor/Model/steam turbine SM ==
  gate : Inport
  Gain : Gain  Gain=(1-initMachineBlocks{SGnum,13}(1))
  Gain1 : Gain  Gain=initMachineBlocks{SGnum,13}(1)
  Stage4 : spsFirstOrderFilterLib/First-Order Filter  FilterType=Lowpass  Tc=initMachineBlocks{SGnum,13}(2)  Ts=Ts  Initialize=on  Vac_Init=[0, 0, T_SG.fb]  Vdc_Init=(1-initMachineBlocks{SGnum,13}(1))*initSG.Pm  PlotResponse=off  FreqRange="[0,  200,  1]"
  Sum : Sum  Inputs=++|
  Tturb : Outport
  wires:
  Stage4/1 -> Sum/2
  Gain1/1 -> Sum/1
  Sum/1 -> Tturb/1
  Gain/1 -> Stage4/1
  gate/1 -> Gain/1, Gain1/1

== system myLibrary/SG/Governor-Turbine/Steam Turbine and Governor/Model/4 mass shaft/1 mass ==
  note: Mass1 = generator rotor simulated in synchronous machine model
  note: Eeach block Mass implements discretized state-space equations
      | of the shaft mass dynamics using trapezoidal method.
      |
      | x(k)= Ad*x(k-1) + Bd*(u(k)+u(k-1))
      |
      | where:
      | x(k) =  State vector = [dw_n             deltat_n   ]'
      | u(k) =  Input vector = [(Ts_n+1 + Tt_n)  deltat_n-1 ]'
      | n    =  Mass number
      |
      | % Discrete state-space matrices
      | Ad = inv(In - Ts/2*A)*(In + Ts/2*A)
      | Bd = inv(In - Ts/2*A)*B*Ts/2
      |
      | where:
      | Continuous state-space matrices:
      | A=[ -K1*D  -K1*K
      |      K2     0   ];
      |
      | B=[ K1  K1*K
      |      0     0];
      |
      | In = eye(2,2)
      | K  = Rigidity (pu)
      | K1 =1/(2*H);  H= inertia  (pu)
      | K2 =N*pi/30;  N=nominal speed of sync. machine (rpm)
  Tt_5-2 : Inport
  dth_gen : Inport  Port=2
  Enable : EnablePort  PropagateVarSize=During execution
  Ground : Ground
  Ground1 : Ground
  Mass2 : Subsystem  mask(Generic rotating mass){H=Ha(1), K=Ka(1), D=Da(1), dth0=dtha(1), N=N, Ts=Ts}
      mask prompts: H "Inertia H (pu)"; K "Rigidity K (pu):"; D "Damping D (pu):"; dth0 "Initial angle deviation delta_theta (rad):"; N "Nominal speed of synchronous machine (rpm):"; Ts "Sample time (s):"
      mask init:
      | %State stpace matrices of the 2-inputs, 3 outputs, 2states system
      | % u1= Ts_k+1 +Tt_k
      | % u2= deltat_k-1
      | % y1= deltat_k
      | % y2= Ts_k
      | % y3= dw
      | % x1= dw
      | % x2= deltat_k
      | 
      | K1=1/2/H;
      | K2=N*pi/30;
      | 
      | A=[ -K1*D  -K1*K 
      |      K2     0   ];
      |  
      | B=[ K1  K1*K 
      |      0     0]; 
      |  
      | %Discretization using trapezoidal method
      | In=eye(2,2);
      | Ad = inv(In - Ts/2*A)*(In + Ts/2*A);
      | Bd = inv(In - Ts/2*A)*B*Ts/2;
  Mux : Mux  Inputs=[3 1]
  Mux1 : Mux  Inputs=[3 1]
  Selector : Selector  InputPortWidth=4  IndexOptions=Index vector (dialog)  Indices=4  OutputSizes=1
  Terminator : Terminator
  Ts_5-2 : Outport  InitialOutput=[0,0,0,0]
  dw_5-2 : Outport  Port=2  InitialOutput=[0,0,0,0]
  Tm_gen : Outport  Port=3
  wires:
  Mux1/1 -> dw_5-2/1
  Mass2/3(dw) -> Mux1/2
  Ground1/1 -> Mux1/1, Mux/1
  Tt_5-2/1 -> Selector/1
  Mux/1 -> Ts_5-2/1
  Selector/1 -> Mass2/2(Tt_n)
  Ground/1 -> Mass2/1(Ts_n+1)
  Mass2/1(deltat_n) -> Terminator/1
  dth_gen/1 -> Mass2/3(deltat_n-1)
  Mass2/2("Ts_n ") -> Mux/2, Tm_gen/1

== system myLibrary/SG/Governor-Turbine/Steam Turbine and Governor/Model/4 mass shaft/2 masses ==
  note: Eeach block Mass implements discretized state-space equations
      | of the shaft mass dynamics using trapezoidal method.
      |
      | x(k)= Ad*x(k-1) + Bd*(u(k)+u(k-1))
      |
      | where:
      | x(k) =  State vector = [dw_n             deltat_n   ]'
      | u(k) =  Input vector = [(Ts_n+1 + Tt_n)  deltat_n-1 ]'
      | n    =  Mass number
      |
      | % Discrete state-space matrices
      | Ad = inv(In - Ts/2*A)*(In + Ts/2*A)
      | Bd = inv(In - Ts/2*A)*B*Ts/2
      |
      | where:
      | Continuous state-space matrices:
      | A=[ -K1*D  -K1*K
      |      K2     0   ];
      |
      | B=[ K1  K1*K
      |      0     0];
      |
      | In = eye(2,2)
      | K  = Rigidity (pu)
      | K1 =1/(2*H);  H= inertia  (pu)
      | K2 =N*pi/30;  N=nominal speed of sync. machine (rpm)
  note: Mass1 = generator rotor simulated in synchronous machine model
  Tt_5-2 : Inport
  dth_gen : Inport  Port=2
  Enable : EnablePort  PropagateVarSize=During execution
  Demux : Demux  Outputs=2
      settings: DisplayOption=none
  Ground : Ground
  Ground1 : Ground
  Mass2 : Subsystem  mask(Generic rotating mass){H=Ha(1), K=Ka(1), D=Da(1), dth0=dtha(1), N=N, Ts=Ts}
      mask prompts: H "Inertia H (pu)"; K "Rigidity K (pu):"; D "Damping D (pu):"; dth0 "Initial angle deviation delta_theta (rad):"; N "Nominal speed of synchronous machine (rpm):"; Ts "Sample time (s):"
      mask init: same as myLibrary/SG/Governor-Turbine/Steam Turbine and Governor/Model/4 mass shaft/1 mass/Mass2
  Mass3 : Subsystem  mask(Generic rotating mass){H=Ha(2), K=Ka(2), D=Da(2), dth0=dtha(2), N=N, Ts=Ts}
      mask prompts: H "Inertia H (pu)"; K "Rigidity K (pu):"; D "Damping D (pu):"; dth0 "Initial angle deviation delta_theta (rad):"; N "Nominal speed of synchronous machine (rpm):"; Ts "Sample time (s):"
      mask init: same as myLibrary/SG/Governor-Turbine/Steam Turbine and Governor/Model/4 mass shaft/1 mass/Mass2
  Mux : Mux  Inputs=[ 2 1 1 ]
  Mux1 : Mux  Inputs=[ 2 1 1 ]
  Selector : Selector  InputPortWidth=4  IndexOptions=Index vector (dialog)  Indices=[3 4]  OutputSizes=1
  Terminator : Terminator
  Ts_5-2 : Outport  InitialOutput=[0,0,0,0]
  dw_5-2 : Outport  Port=2  InitialOutput=[0,0,0,0]
  Tm_gen : Outport  Port=3
  wires:
  Mass2/3(dw) -> Mux1/3
  Mass3/3(dw) -> Mux1/2
  Mux1/1 -> dw_5-2/1
  Ground1/1 -> Mux1/1, Mux/1
  Demux/1 -> Mass3/2(Tt_n)
  Tt_5-2/1 -> Selector/1
  Selector/1 -> Demux/1
  Mux/1 -> Ts_5-2/1
  Mass3/2("Ts_n ") -> Mux/2, Mass2/1(Ts_n+1)
  Mass3/1(deltat_n) -> Terminator/1
  Ground/1 -> Mass3/1(Ts_n+1)
  Demux/2 -> Mass2/2(Tt_n)
  Mass2/1(deltat_n) -> Mass3/3(deltat_n-1)
  dth_gen/1 -> Mass2/3(deltat_n-1)
  Mass2/2("Ts_n ") -> Mux/3, Tm_gen/1

== system myLibrary/SG/Governor-Turbine/Steam Turbine and Governor/Model/4 mass shaft/3 masses ==
  note: Eeach block Mass implements discretized state-space equations
      | of the shaft mass dynamics using trapezoidal method.
      |
      | x(k)= Ad*x(k-1) + Bd*(u(k)+u(k-1))
      |
      | where:
      | x(k) =  State vector = [dw_n             deltat_n   ]'
      | u(k) =  Input vector = [(Ts_n+1 + Tt_n)  deltat_n-1 ]'
      | n    =  Mass number
      |
      | % Discrete state-space matrices
      | Ad = inv(In - Ts/2*A)*(In + Ts/2*A)
      | Bd = inv(In - Ts/2*A)*B*Ts/2
      |
      | where:
      | Continuous state-space matrices:
      | A=[ -K1*D  -K1*K
      |      K2     0   ];
      |
      | B=[ K1  K1*K
      |      0     0];
      |
      | In = eye(2,2)
      | K  = Rigidity (pu)
      | K1 =1/(2*H);  H= inertia  (pu)
      | K2 =N*pi/30;  N=nominal speed of sync. machine (rpm)
  note: Mass1 = generator rotor simulated in synchronous machine model
  Tt_5-2 : Inport
  dth_gen : Inport  Port=2
  Enable : EnablePort  PropagateVarSize=During execution
  Demux : Demux  Outputs=3
      settings: DisplayOption=none
  Ground : Ground
  Ground1 : Ground
  Mass2 : Subsystem  mask(Generic rotating mass){H=Ha(1), K=Ka(1), D=Da(1), dth0=dtha(1), N=N, Ts=Ts}
      mask prompts: H "Inertia H (pu)"; K "Rigidity K (pu):"; D "Damping D (pu):"; dth0 "Initial angle deviation delta_theta (rad):"; N "Nominal speed of synchronous machine (rpm):"; Ts "Sample time (s):"
      mask init: same as myLibrary/SG/Governor-Turbine/Steam Turbine and Governor/Model/4 mass shaft/1 mass/Mass2
  Mass3 : Subsystem  mask(Generic rotating mass){H=Ha(2), K=Ka(2), D=Da(2), dth0=dtha(2), N=N, Ts=Ts}
      mask prompts: H "Inertia H (pu)"; K "Rigidity K (pu):"; D "Damping D (pu):"; dth0 "Initial angle deviation delta_theta (rad):"; N "Nominal speed of synchronous machine (rpm):"; Ts "Sample time (s):"
      mask init: same as myLibrary/SG/Governor-Turbine/Steam Turbine and Governor/Model/4 mass shaft/1 mass/Mass2
  Mass4 : Subsystem  mask(Generic rotating mass){H=Ha(3), K=Ka(3), D=Da(3), dth0=dtha(3), N=N, Ts=Ts}
      mask prompts: H "Inertia H (pu)"; K "Rigidity K (pu):"; D "Damping D (pu):"; dth0 "Initial angle deviation delta_theta (rad):"; N "Nominal speed of synchronous machine (rpm):"; Ts "Sample time (s):"
      mask init: same as myLibrary/SG/Governor-Turbine/Steam Turbine and Governor/Model/4 mass shaft/1 mass/Mass2
  Mux : Mux
  Mux1 : Mux
  Selector : Selector  InputPortWidth=4  IndexOptions=Index vector (dialog)  Indices=[2 3 4]  OutputSizes=1
  Terminator : Terminator
  Ts_5-2 : Outport  InitialOutput=[0,0,0,0]
  dw_5-2 : Outport  Port=2  InitialOutput=[0,0,0,0]
  Tm_gen : Outport  Port=3
  wires:
  Mass2/3(dw) -> Mux1/4
  Mux1/1 -> dw_5-2/1
  Ground1/1 -> Mux1/1, Mux/1
  Mux/1 -> Ts_5-2/1
  Mass3/3(dw) -> Mux1/3
  Mass4/3(dw) -> Mux1/2
  Mass4/2("Ts_n ") -> Mux/2, Mass3/1(Ts_n+1)
  Mass3/1(deltat_n) -> Mass4/3(deltat_n-1)
  Mass2/1(deltat_n) -> Mass3/3(deltat_n-1)
  Demux/3 -> Mass2/2(Tt_n)
  Demux/2 -> Mass3/2(Tt_n)
  Demux/1 -> Mass4/2(Tt_n)
  Ground/1 -> Mass4/1(Ts_n+1)
  Mass4/1(deltat_n) -> Terminator/1
  dth_gen/1 -> Mass2/3(deltat_n-1)
  Mass2/2("Ts_n ") -> Tm_gen/1, Mux/4
  Selector/1 -> Demux/1
  Tt_5-2/1 -> Selector/1
  Mass3/2("Ts_n ") -> Mux/3, Mass2/1(Ts_n+1)

== system myLibrary/SG/Governor-Turbine/Steam Turbine and Governor/Model/4 mass shaft/4 masses ==
  note: Eeach block Mass implements discretized state-space equations
      | of the shaft mass dynamics using trapezoidal method.
      |
      | x(k)= Ad*x(k-1) + Bd*(u(k)+u(k-1))
      |
      | where:
      | x(k) =  State vector = [dw_n             deltat_n   ]'
      | u(k) =  Input vector = [(Ts_n+1 + Tt_n)  deltat_n-1 ]'
      | n    =  Mass number
      |
      | % Discrete state-space matrices
      | Ad = inv(In - Ts/2*A)*(In + Ts/2*A)
      | Bd = inv(In - Ts/2*A)*B*Ts/2
      |
      | where:
      | Continuous state-space matrices:
      | A=[ -K1*D  -K1*K
      |      K2     0   ];
      |
      | B=[ K1  K1*K
      |      0     0];
      |
      | In = eye(2,2)
      | K  = Rigidity (pu)
      | K1 =1/(2*H);  H= inertia  (pu)
      | K2 =N*pi/30;  N=nominal speed of sync. machine (rpm)
  note: Mass1 = generator rotor simulated in synchronous machine model
  Tt_5-2 : Inport
  dth_gen : Inport  Port=2
  Enable : EnablePort  PropagateVarSize=During execution
  Demux : Demux
      settings: DisplayOption=none
  Ground : Ground
  Mass2 : Subsystem  mask(Generic rotating mass){H=Ha(1), K=Ka(1), D=Da(1), dth0=initSG.delta2, N=N, Ts=Ts}
      mask prompts: H "Inertia H (pu)"; K "Rigidity K (pu):"; D "Damping D (pu):"; dth0 "Initial angle deviation delta_theta (rad):"; N "Nominal speed of synchronous machine (rpm):"; Ts "Sample time (s):"
      mask init: same as myLibrary/SG/Governor-Turbine/Steam Turbine and Governor/Model/4 mass shaft/1 mass/Mass2
  Mass3 : Subsystem  mask(Generic rotating mass){H=Ha(2), K=Ka(2), D=Da(2), dth0=initSG.delta3, N=N, Ts=Ts}
      mask prompts: H "Inertia H (pu)"; K "Rigidity K (pu):"; D "Damping D (pu):"; dth0 "Initial angle deviation delta_theta (rad):"; N "Nominal speed of synchronous machine (rpm):"; Ts "Sample time (s):"
      mask init: same as myLibrary/SG/Governor-Turbine/Steam Turbine and Governor/Model/4 mass shaft/1 mass/Mass2
  Mass4 : Subsystem  mask(Generic rotating mass){H=Ha(3), K=Ka(3), D=Da(3), dth0=initSG.delta4, N=N, Ts=Ts}
      mask prompts: H "Inertia H (pu)"; K "Rigidity K (pu):"; D "Damping D (pu):"; dth0 "Initial angle deviation delta_theta (rad):"; N "Nominal speed of synchronous machine (rpm):"; Ts "Sample time (s):"
      mask init: same as myLibrary/SG/Governor-Turbine/Steam Turbine and Governor/Model/4 mass shaft/1 mass/Mass2
  Mass5 : Subsystem  mask(Generic rotating mass){H=Ha(4), K=Ka(4), D=Da(4), dth0=initSG.delta5, N=N, Ts=Ts}
      mask prompts: H "Inertia H (pu)"; K "Rigidity K (pu):"; D "Damping D (pu):"; dth0 "Initial angle deviation delta_theta (rad):"; N "Nominal speed of synchronous machine (rpm):"; Ts "Sample time (s):"
      mask init: same as myLibrary/SG/Governor-Turbine/Steam Turbine and Governor/Model/4 mass shaft/1 mass/Mass2
  Mux : Mux
  Mux1 : Mux
  Terminator : Terminator
  Ts_5-2 : Outport  InitialOutput=[0,0,0,0]
  dw_5-2 : Outport  Port=2  InitialOutput=[0,0,0,0]
  Tm_gen : Outport  Port=3
  wires:
  Mass2/3(dw) -> Mux1/4
  Mass3/3(dw) -> Mux1/3
  Mux1/1 -> dw_5-2/1
  Mass4/3(dw) -> Mux1/2
  Mass5/3(dw) -> Mux1/1
  Mux/1 -> Ts_5-2/1
  Mass5/1(deltat_n) -> Terminator/1
  Ground/1 -> Mass5/1(Ts_n+1)
  Demux/1 -> Mass5/2(Tt_n)
  Demux/2 -> Mass4/2(Tt_n)
  Demux/3 -> Mass3/2(Tt_n)
  Demux/4 -> Mass2/2(Tt_n)
  Mass2/1(deltat_n) -> Mass3/3(deltat_n-1)
  Mass3/1(deltat_n) -> Mass4/3(deltat_n-1)
  Mass4/1(deltat_n) -> Mass5/3(deltat_n-1)
  Mass5/2("Ts_n ") -> Mux/1, Mass4/1(Ts_n+1)
  Mass4/2("Ts_n ") -> Mux/2, Mass3/1(Ts_n+1)
  Mass3/2("Ts_n ") -> Mux/3, Mass2/1(Ts_n+1)
  Tt_5-2/1 -> Demux/1
  dth_gen/1 -> Mass2/3(deltat_n-1)
  Mass2/2("Ts_n ") -> Mux/4, Tm_gen/1

== system myLibrary/SG/Governor-Turbine/Steam Turbine and Governor/Model/steam turbine MM/Stage 1 ==
  In1 : Inport
  Constant4 : Constant  Value=Ta(1)~=0  SampleTime=Ts
  Stage1 : Subsystem  TreatAsAtomicUnit=on
  Switch : Switch  Threshold=0.5  SaturateOnIntegerOverflow=off
  Out1 : Outport
  wires:
  Constant4/1 -> Stage1/Enable, Switch/2
  In1/1 -> Stage1/1(In1), Switch/3
  Stage1/1(Out1) -> Switch/1
  Switch/1 -> Out1/1

== system myLibrary/SG/Governor-Turbine/Steam Turbine and Governor/Model/steam turbine MM/Stage 2  ==
  In1 : Inport
  Constant3 : Constant  Value=Ta(2)~=0  SampleTime=Ts
  Stage2 : Subsystem  TreatAsAtomicUnit=on
  Switch1 : Switch  Threshold=0.5  SaturateOnIntegerOverflow=off
  Out1 : Outport
  wires:
  Stage2/1(Out1) -> Switch1/1
  Constant3/1 -> Stage2/Enable, Switch1/2
  Switch1/1 -> Out1/1
  In1/1 -> Stage2/1(In1), Switch1/3

== system myLibrary/SG/Governor-Turbine/Steam Turbine and Governor/Model/steam turbine MM/Stage 3 ==
  In1 : Inport
  Constant2 : Constant  Value=Ta(3)~=0  SampleTime=Ts
  Stage3 : Subsystem  TreatAsAtomicUnit=on
  Switch2 : Switch  Threshold=0.5  SaturateOnIntegerOverflow=off
  Out1 : Outport
  wires:
  Stage3/1(Out1) -> Switch2/1
  Constant2/1 -> Stage3/Enable, Switch2/2
  Switch2/1 -> Out1/1
  In1/1 -> Stage3/1(In1), Switch2/3

== system myLibrary/SG/Governor-Turbine/Steam Turbine and Governor/Model/steam turbine MM/Stage 4 ==
  In1 : Inport
  Constant1 : Constant  Value=Ta(4)~=0  SampleTime=Ts
  Stage4 : Subsystem  TreatAsAtomicUnit=on
  Switch3 : Switch  Threshold=0.5  SaturateOnIntegerOverflow=off
  Out1 : Outport
  wires:
  Stage4/1(Out1) -> Switch3/1
  Constant1/1 -> Stage4/Enable, Switch3/2
  In1/1 -> Stage4/1(In1), Switch3/3
  Switch3/1 -> Out1/1

== system myLibrary/SG_step/Governor-Turbine/Steam Turbine and Governor/Model/4 mass shaft/1 mass ==
  note: Mass1 = generator rotor simulated in synchronous machine model
  note: Eeach block Mass implements discretized state-space equations
      | of the shaft mass dynamics using trapezoidal method.
      |
      | x(k)= Ad*x(k-1) + Bd*(u(k)+u(k-1))
      |
      | where:
      | x(k) =  State vector = [dw_n             deltat_n   ]'
      | u(k) =  Input vector = [(Ts_n+1 + Tt_n)  deltat_n-1 ]'
      | n    =  Mass number
      |
      | % Discrete state-space matrices
      | Ad = inv(In - Ts/2*A)*(In + Ts/2*A)
      | Bd = inv(In - Ts/2*A)*B*Ts/2
      |
      | where:
      | Continuous state-space matrices:
      | A=[ -K1*D  -K1*K
      |      K2     0   ];
      |
      | B=[ K1  K1*K
      |      0     0];
      |
      | In = eye(2,2)
      | K  = Rigidity (pu)
      | K1 =1/(2*H);  H= inertia  (pu)
      | K2 =N*pi/30;  N=nominal speed of sync. machine (rpm)
  Tt_5-2 : Inport
  dth_gen : Inport  Port=2
  Enable : EnablePort  PropagateVarSize=During execution
  Ground : Ground
  Ground1 : Ground
  Mass2 : Subsystem  mask(Generic rotating mass){H=Ha(1), K=Ka(1), D=Da(1), dth0=dtha(1), N=N, Ts=Ts}
      mask prompts: H "Inertia H (pu)"; K "Rigidity K (pu):"; D "Damping D (pu):"; dth0 "Initial angle deviation delta_theta (rad):"; N "Nominal speed of synchronous machine (rpm):"; Ts "Sample time (s):"
      mask init: same as myLibrary/SG/Governor-Turbine/Steam Turbine and Governor/Model/4 mass shaft/1 mass/Mass2
  Mux : Mux  Inputs=[3 1]
  Mux1 : Mux  Inputs=[3 1]
  Selector : Selector  InputPortWidth=4  IndexOptions=Index vector (dialog)  Indices=4  OutputSizes=1
  Terminator : Terminator
  Ts_5-2 : Outport  InitialOutput=[0,0,0,0]
  dw_5-2 : Outport  Port=2  InitialOutput=[0,0,0,0]
  Tm_gen : Outport  Port=3
  wires:
  Mux1/1 -> dw_5-2/1
  Mass2/3(dw) -> Mux1/2
  Ground1/1 -> Mux1/1, Mux/1
  Tt_5-2/1 -> Selector/1
  Mux/1 -> Ts_5-2/1
  Selector/1 -> Mass2/2(Tt_n)
  Ground/1 -> Mass2/1(Ts_n+1)
  Mass2/1(deltat_n) -> Terminator/1
  dth_gen/1 -> Mass2/3(deltat_n-1)
  Mass2/2("Ts_n ") -> Mux/2, Tm_gen/1
